simulink model "out_put"  (R2019b)
settings: Solver=ode1  StartTime=ts  StopTime=10.0  FixedStep=dt  RelTol=1e-3
(part 1 of 3)
settings Model: Creator=a4327  LastModifiedBy=a4327
settings DataIOCC: SaveOutput=off  SaveTime=off
settings OptimizationCC: DefaultParameterBehavior=Inlined

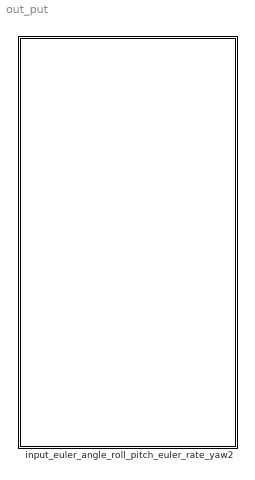
== system out_put ==
  input_euler_angle_roll_pitch_euler_rate_yaw2 : Subsystem
      mask help: Simulink:masks:GenSFuncDesc_MD
      mask Help: eval('feval(''rtwprivate'',''rtwhelpview'',''rtw_sfcn_block'')');
